simulink model "simulink_ex_4"  (R2021a)
settings: Solver=VariableStepAuto  StartTime=0.0  StopTime=50000  RelTol=1e-3
settings Model: Creator=HanO  LastModifiedBy=HanO

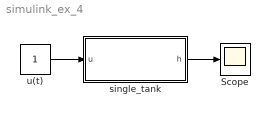
== system simulink_ex_4 ==
  Scope : Scope
  single_tank : Subsystem  mask{a=0.1, AA=10, k=0.5, Cd=0.1, g=9.81, h0=5}
      mask prompts: a "Tiết diện van xả a ="; AA "Tiết diện ngang bồn chứa A ="; k "Hệ số tỉ lệ công suất máy bơm k ="; Cd "Hệ số xả Cd ="; g "Gia tốc trọng trường g ="; h0 "Chiều cao mực nước ban đầu h0 ="
  u(t) : Constant
  wires:
  u(t)/1 -> single_tank/1(u)
  single_tank/1(h) -> Scope/1

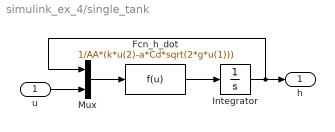
== system simulink_ex_4/single_tank ==
  u : Inport
  Fcn_h_dot : Fcn  Expr=1/AA*(k*u(2)-a*Cd*sqrt(2*g*u(1)))
  Integrator : Integrator  InitialCondition=h0
  Mux : Mux  Inputs=2
  h : Outport
  wires:
  Fcn_h_dot/1 -> Integrator/1
  u/1 -> Mux/2
  Mux/1 -> Fcn_h_dot/1
  Integrator/1 -> Mux/1, h/1
